simulink model "pr642_PLL_linear_model"  (R2018b)
settings: Solver=VariableStepAuto  StartTime=0.0  StopTime=1  RelTol=1e-3
libraries: simulink x1
settings Model: Creator=Григорий Фокин  LastModifiedBy=Григорий Фокин

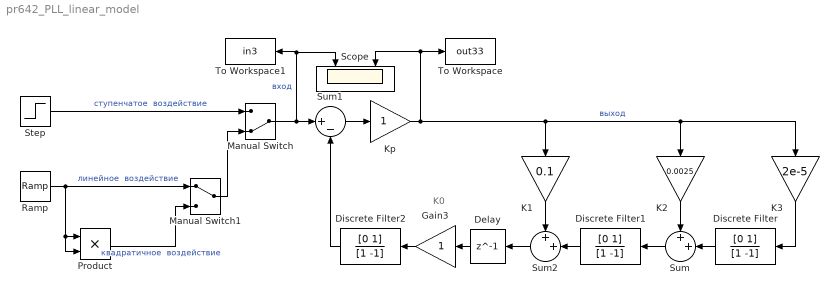
== system pr642_PLL_linear_model ==
  note: K0
  Delay : Delay  DelayLength=1  InitialCondition=0
  Discrete Filter : DiscreteFilter  Numerator=[0 1]  Denominator=[1 -1]  SampleTime=1/1000
  Discrete Filter1 : DiscreteFilter  Numerator=[0 1]  Denominator=[1 -1]  SampleTime=1/1000
  Discrete Filter2 : DiscreteFilter  Numerator=[0 1]  Denominator=[1 -1]  SampleTime=1/1000
  Gain3 : Gain
  K1 : Gain  Gain=0.1
  K2 : Gain  Gain=0.0025
  K3 : Gain  Gain=2e-5
  Kp : Gain
  Manual Switch : ManualSwitch  CurrentSetting=0
  Manual Switch1 : ManualSwitch
  Product : Product
  Ramp : simulink/Sources/Ramp  slope=2  start=0.2  InitialOutput=0
  Scope : Scope  NumInputPorts=2
  Step : Step  Time=0.2  SampleTime=1/1000
  Sum : Sum  Inputs=++|
  Sum1 : Sum  Inputs=|+-
  Sum2 : Sum  Inputs=++|
  To Workspace : ToWorkspace  VariableName=out33  SaveFormat=Timeseries  SampleTime=-1
  To Workspace1 : ToWorkspace  VariableName=in3  SaveFormat=Timeseries  SampleTime=-1
  wires:
  Step/1 -> Manual Switch/1  "ступенчатое  воздействие"
  Ramp/1 -> Manual Switch1/1, Product/2, Product/1  "линейное  воздействие"
  Product/1 -> Manual Switch1/2  "квадратичное  воздействие"
  Manual Switch/1 -> Scope/1, To Workspace1/1, Sum1/1  "вход"
  K3/1 -> Discrete Filter/1
  Discrete Filter/1 -> Sum/2
  K2/1 -> Sum/1
  K1/1 -> Sum2/1
  Discrete Filter1/1 -> Sum2/2
  Sum/1 -> Discrete Filter1/1
  Sum2/1 -> Delay/1
  Delay/1 -> Gain3/1
  Gain3/1 -> Discrete Filter2/1
  Discrete Filter2/1 -> Sum1/2
  Sum1/1 -> Kp/1
  Kp/1 -> Scope/2, To Workspace/1, K3/1, K2/1, K1/1  "выход"
  Manual Switch1/1 -> Manual Switch/2
